simulink model "nms_3Dmodel_inv_wAnkleCPG"  (R2016b)
settings: Solver=ode3  StartTime=0.0  StopTime=tend  FixedStep=ts  RelTol=1e-3  EnableMultiTasking=on
InitFcn:
  | runScripts_inv;
values from neighbouring files (symbols this model uses):
  c = 0.05    [IID_nms_MechInit.m]    (also in nms_MechInit.m)
  c_jointstop = 0.3 / (pi/180)    (= 17.1887338539)    [IID_nms_MechInit.m]    (also in nms_MechInit.m)
  CPG_On = 1    [setCPGPar.m]    (also in setCPGPar_inv.m)
  CtrlPar_FP = [alpha0 alpha_cd alpha_cv]    [setCtrlPar.m]
  CtrlPar_FP_R = [R_hipR0 R_hipR_cd R_hipR_cv]    [setCtrlPar.m]
  CtrlPar_LL = l_clr    [setCtrlPar.m]
  CtrlPar_St = [StPreStim St_M1 St_M2 St_M3 St_M4 St_M5 St_M11]    [setCtrlPar.m]
  CtrlPar_St_R = [R_StPreStim R_St_M1 R_St_M3 R_St_M4]    [setCtrlPar.m]
  CtrlPar_Sw = [SwPreStim SwPhasePari SwPhaseParii SwCtrlPar_H SwCtrlPar_A      SwCtrlPar_Ki SwCtrlPar_Kii SwCtrlPar_Kiii SwCtrlPar_StP]    [setCtrlPar.m]
  CtrlPar_Sw_R = [R_SwPreStim R_Sw_M6]    [setCtrlPar.m]
  CtrlPar_theta0 = parBlCtrl(1)      *1*pi/180    [setCtrlPar.m]
  CtrlPar_Tr = [Tr_St_sup Tr_Sw]    [setCtrlPar.m]
  CtrlPar_Tr_R = [R_Tr_St_sup R_Tr_Sw]    [setCtrlPar.m]
  eref = 0.04    [IID_nms_MechInit.m]    (also in nms_MechInit.m)
  FmaxBFSH = 350    [nms_MechInit.m]
  FmaxGAS = 1500    [IID_nms_MechInit.m]    (also in nms_MechInit.m)
  FmaxGLU = 1500    [IID_nms_MechInit.m]    (also in nms_MechInit.m)
  FmaxHAB = 3000    [nms_MechInit.m]
  FmaxHAD = 4500    [nms_MechInit.m]
  FmaxHAM = 3000    [IID_nms_MechInit.m]    (also in nms_MechInit.m)
  FmaxHFL = 2000    [IID_nms_MechInit.m]    (also in nms_MechInit.m)
  FmaxRF = 1200    [nms_MechInit.m]
  FmaxSOL = 4000    [IID_nms_MechInit.m]    (also in nms_MechInit.m)
  FmaxTA = 800    [IID_nms_MechInit.m]    (also in nms_MechInit.m)
  FmaxVAS = 6000    [IID_nms_MechInit.m]    (also in nms_MechInit.m)
  init_a_tgt = 70*pi/180    (= 1.2217304764)    [setInitPar.m]
  init_a_tgtR = 90*pi/180    (= 1.57079632679)    [setInitPar.m]
  K = 5    [IID_nms_MechInit.m]    (also in nms_MechInit.m)
  leg_l = [D12_T D12_S]    [nms_MechInit.m]
  LongDelay = 0.020    (= 0.02)    [IID_setCtrlPar.m]    (also in nms_MechInit.m = 0.01)
  LongLoopDelay = 0.030    (= 0.03)    [nms_MechInit.m]
  loptBFSH = 0.12    [nms_MechInit.m]
  loptGAS = 0.05    [IID_nms_MechInit.m]    (also in nms_MechInit.m)
  loptGLU = 0.11    [IID_nms_MechInit.m]    (also in nms_MechInit.m)
  loptHAB = 0.09    [nms_MechInit.m]
  loptHAD = 0.10    (= 0.1)    [nms_MechInit.m]
  loptHAM = 0.10    (= 0.1)    [IID_nms_MechInit.m]    (also in nms_MechInit.m)
  loptHFL = 0.11    [IID_nms_MechInit.m]    (also in nms_MechInit.m)
  loptRF = 0.08    [nms_MechInit.m]
  loptSOL = 0.04    [IID_nms_MechInit.m]    (also in nms_MechInit.m)
  loptTA = 0.06    [IID_nms_MechInit.m]    (also in nms_MechInit.m)
  loptVAS = 0.08    [IID_nms_MechInit.m]    (also in nms_MechInit.m)
  lslackBFSH = 0.10    (= 0.1)    [nms_MechInit.m]
  lslackGAS = 0.40    (= 0.4)    [IID_nms_MechInit.m]    (also in nms_MechInit.m)
  lslackGLU = 0.13    [IID_nms_MechInit.m]    (also in nms_MechInit.m)
  lslackHAB = 0.07    [nms_MechInit.m]
  lslackHAD = 0.18    [nms_MechInit.m]
  lslackHAM = 0.31    [IID_nms_MechInit.m]    (also in nms_MechInit.m)
  lslackHFL = 0.10    (= 0.1)    [IID_nms_MechInit.m]    (also in nms_MechInit.m)
  lslackRF = 0.35    [nms_MechInit.m]
  lslackSOL = 0.26    [IID_nms_MechInit.m]    (also in nms_MechInit.m)
  lslackTA = 0.24    [IID_nms_MechInit.m]    (also in nms_MechInit.m)
  lslackVAS = 0.23    [IID_nms_MechInit.m]    (also in nms_MechInit.m)
  massBFSH = 2    [nms_MechInit.m]
  massGAS = 0.45    [IID_nms_MechInit.m]    (also in nms_MechInit.m)
  massGLU = 1.4    [IID_nms_MechInit.m]    (also in nms_MechInit.m)
  massHAB = 1.145    [nms_MechInit.m]
  massHAD = 1.91    [nms_MechInit.m]
  massHAM = 1.82    [IID_nms_MechInit.m]    (also in nms_MechInit.m)
  massHFL = 1.87    [IID_nms_MechInit.m]    (also in nms_MechInit.m)
  massRF = 1    [nms_MechInit.m]
  massSOL = 1.36    [IID_nms_MechInit.m]    (also in nms_MechInit.m)
  massTA = 0.29    [IID_nms_MechInit.m]    (also in nms_MechInit.m)
  massVAS = 2.91    [IID_nms_MechInit.m]    (also in nms_MechInit.m)
  MidDelay = 0.010    (= 0.01)    [IID_setCtrlPar.m]    (also in nms_MechInit.m = 0.005)
  N = 1.5    [IID_nms_MechInit.m]    (also in cmaes_parfor.m = size(x,1); nms_MechInit.m)
  phi12_LowLimit = 70*pi/180    (= 1.2217304764)    [IID_nms_MechInit.m]    (also in nms_MechInit.m)
  phi12_UpLimit = 130*pi/180    (= 2.26892802759)    [IID_nms_MechInit.m]    (also in nms_MechInit.m)
  phi23_UpLimit = 175*pi/180    (= 3.05432619099)    [IID_nms_MechInit.m]    (also in nms_MechInit.m)
  phi34_UpLimit = 230*pi/180    (= 4.01425727959)    [IID_nms_MechInit.m]    (also in nms_MechInit.m)
  phi34R_LowLimit = -15*pi/180    (= -0.261799387799)    [nms_MechInit.m]
  phi34R_UpLimit = 50*pi/180    (= 0.872664625997)    [nms_MechInit.m]
  phimaxGASa = 110*pi/180    (= 1.91986217719)    [IID_nms_MechInit.m]    (also in nms_MechInit.m = 1.74532925199)
  phimaxGASk = 140*pi/180    (= 2.44346095279)    [IID_nms_MechInit.m]    (also in nms_MechInit.m)
  phimaxRFk = 165*pi/180    (= 2.87979326579)    [nms_MechInit.m]
  phimaxSOL = 110*pi/180    (= 1.91986217719)    [IID_nms_MechInit.m]    (also in nms_MechInit.m = 1.74532925199)
  phimaxTA = 80*pi/180    (= 1.3962634016)    [IID_nms_MechInit.m]    (also in nms_MechInit.m)
  phimaxVAS = 165*pi/180    (= 2.87979326579)    [IID_nms_MechInit.m]    (also in nms_MechInit.m)
  phirefBFSH = 160*pi/180    (= 2.79252680319)    [nms_MechInit.m]
  phirefGASa = 80*pi/180    (= 1.3962634016)    [IID_nms_MechInit.m]    (also in nms_MechInit.m)
  phirefGASk = 165*pi/180    (= 2.87979326579)    [IID_nms_MechInit.m]    (also in nms_MechInit.m)
  phirefGLU = 150*pi/180    (= 2.61799387799)    [IID_nms_MechInit.m]    (also in nms_MechInit.m = 2.09439510239)
  phirefHAB = 10*pi/180    (= 0.174532925199)    [nms_MechInit.m]
  phirefHAD = 15*pi/180    (= 0.261799387799)    [nms_MechInit.m]
  phirefHAMh = 155*pi/180    (= 2.70526034059)    [IID_nms_MechInit.m]    (also in nms_MechInit.m = 2.61799387799)
  phirefHAMk = 180*pi/180    (= 3.14159265359)    [IID_nms_MechInit.m]    (also in nms_MechInit.m)
  phirefHFL = 180*pi/180    (= 3.14159265359)    [IID_nms_MechInit.m]    (also in nms_MechInit.m = 2.79252680319)
  phirefRFh = 170*pi/180    (= 2.96705972839)    [nms_MechInit.m]
  phirefRFk = 125*pi/180    (= 2.18166156499)    [nms_MechInit.m]
  phirefSOL = 80*pi/180    (= 1.3962634016)    [IID_nms_MechInit.m]    (also in nms_MechInit.m = 1.57079632679)
  phirefTA = 110*pi/180    (= 1.91986217719)    [IID_nms_MechInit.m]    (also in nms_MechInit.m)
  phirefVAS = 125*pi/180    (= 2.18166156499)    [IID_nms_MechInit.m]    (also in nms_MechInit.m = 2.09439510239)
  phiScaleGASa = acos(rGASamin/rGASamax)/(phiminGASa-phimaxGASa)    [nms_MechInit.m]
  phiScaleGASk = acos(rGASkmin/rGASkmax)/(phiminGASk-phimaxGASk)    [nms_MechInit.m]
  phiScaleRFk = acos(rRFkmin/rRFkmax)/(phiminRFk-phimaxRFk)    [nms_MechInit.m]
  phiScaleSOL = acos(rSOLmin/rSOLmax)/(phiminSOL-phimaxSOL)    [nms_MechInit.m]
  phiScaleTA = acos(rTAmin/rTAmax)/(phiminTA-phimaxTA)    [nms_MechInit.m]
  phiScaleVAS = acos(rVASmin/rVASmax)/(phiminVAS-phimaxVAS)    [nms_MechInit.m]
  rBFSH = 0.04    [nms_MechInit.m]
  rGASamax = 0.06    [nms_MechInit.m]
  rGASkmax = 0.05    [nms_MechInit.m]
  rGLU = 0.10    (= 0.1)    [IID_nms_MechInit.m]    (also in nms_MechInit.m = 0.08)
  rHAB = 0.06    [nms_MechInit.m]
  rHAD = 0.03    [nms_MechInit.m]
  rHAMh = 0.08    [IID_nms_MechInit.m]    (also in nms_MechInit.m)
  rHAMk = 0.05    [IID_nms_MechInit.m]    (also in nms_MechInit.m)
  rHFL = 0.10    (= 0.1)    [IID_nms_MechInit.m]    (also in nms_MechInit.m = 0.08)
  rhoBFSH = 0.7    [nms_MechInit.m]
  rhoGASa = 0.7    [IID_nms_MechInit.m]    (also in nms_MechInit.m)
  rhoGASk = 0.7    [IID_nms_MechInit.m]    (also in nms_MechInit.m)
  rhoGLU = 0.5    [IID_nms_MechInit.m]    (also in nms_MechInit.m)
  rhoHAB = 0.7    [nms_MechInit.m]
  rhoHAD = 1    [nms_MechInit.m]
  rhoHAMh = 0.7    [IID_nms_MechInit.m]    (also in nms_MechInit.m = 0.5)
  rhoHAMk = 0.7    [IID_nms_MechInit.m]    (also in nms_MechInit.m = 0.5)
  rhoHFL = 0.5    [IID_nms_MechInit.m]    (also in nms_MechInit.m)
  rhoRFh = 0.3    [nms_MechInit.m]
  rhoRFk = 0.5    [nms_MechInit.m]
  rhoSOL = 0.5    [IID_nms_MechInit.m]    (also in nms_MechInit.m)
  rhoTA = 0.7    [IID_nms_MechInit.m]    (also in nms_MechInit.m)
  ... (+55 more)
libraries: simulink_extras x30, nmc x30, simulink x22, NMCCPG_Library x13, powerlib_meascontrol x5
(part 6 of 12)

== system nms_3Dmodel_inv_wAnkleCPG/NMC Model/Muscle Actuation Layer/R HFL ==
  note: Excitation Contraction Coupling
  note: HFL Muscle-Tendon Dynamics
  STIM : Inport
  lmtc [m] : Inport  Port=2
  1 : Product  Inputs=**  SaturateOnIntegerOverflow=on  InputSameDT=on  OutDataTypeStr=Inherit: Same as first input
  1/lslack : Gain  Gain=1/lslackHFL  SaturateOnIntegerOverflow=on  OutDataTypeStr=Inherit: Same as input  ParamDataTypeStr=Inherit: Same as input
  2 : Product  Inputs=***  SaturateOnIntegerOverflow=on  InputSameDT=on  OutDataTypeStr=Inherit: Same as first input
  BE force-length relation : Subsystem
  CE force-length relation : Subsystem
  CE inverse force-velocity relation : Subsystem
  Constant : Constant  Value=lslackHFL
  ECC TransferFcn : simulink_extras/Additional Linear/Transfer Fcn (with initial outputs)  N=[1]  D="[tau  1]"  Y0=preA  U0=0
      settings: AttributesFormatString=pre-activation: %<Y0>
  Fmax : Gain  Gain=FmaxHFL  SaturateOnIntegerOverflow=on  OutDataTypeStr=Inherit: Same as input  ParamDataTypeStr=Inherit: Same as input
  Fmax1 : Gain  Gain=FmaxHFL  SaturateOnIntegerOverflow=on  OutDataTypeStr=Inherit: Same as input  ParamDataTypeStr=Inherit: Same as input
  Fv = Fse / (A*Fce) : Product  Inputs=*/  SaturateOnIntegerOverflow=on  InputSameDT=on  OutDataTypeStr=Inherit: Same as first input
  Integrator : Integrator  InitialConditionSource=external  LowerSaturationLimit=0.05  ZeroCross=off
  PE force-length relation : Subsystem
  SE force-length relation : Subsystem
  Sum : Sum  Inputs=|+-  SaturateOnIntegerOverflow=on  InputSameDT=on  OutDataTypeStr=Inherit: Same as first input
  Sum2 : Sum  Inputs=|-+  SaturateOnIntegerOverflow=on  InputSameDT=on  OutDataTypeStr=Inherit: Same as first input
  Sum3 : Sum  SaturateOnIntegerOverflow=on  InputSameDT=on  OutDataTypeStr=Inherit: Same as first input
  Sum4 : Sum  SaturateOnIntegerOverflow=on  InputSameDT=on  OutDataTypeStr=Inherit: Same as first input
  lce/lopt : Gain  Gain=1/loptHFL  SaturateOnIntegerOverflow=on  OutDataTypeStr=Inherit: Same as input  ParamDataTypeStr=Inherit: Same as input
  vmax*lopt : Gain  Gain=vmaxHFL*loptHFL  SaturateOnIntegerOverflow=on  OutDataTypeStr=Inherit: Same as input  ParamDataTypeStr=Inherit: Same as input
  Fmtc : Outport  InitialOutput=0
  Lce : Outport  Port=2  InitialOutput=0
  Vce : Outport  Port=3  InitialOutput=0
  A : Outport  Port=4  InitialOutput=0
  Fac : Outport  Port=5  InitialOutput=0
  wires:
  Fmax1/1 -> Fac/1
  2/1 -> Fmax1/1
  ECC TransferFcn/1 -> 1/2, A/1, 2/2  "A"
  STIM/1 -> ECC TransferFcn/1
  CE inverse force-velocity relation/1(v[vmax]) -> vmax*lopt/1
  Sum3/1 -> Fv = Fse / (A*Fce)/2
  BE force-length relation/1(fbe [Fmax]) -> Sum4/2  "Fbe"
  1/1 -> Sum3/2
  PE force-length relation/1(fpe [Fmax]) -> Sum3/1  "Fpe"
  Sum4/1 -> Fv = Fse / (A*Fce)/1
  CE force-length relation/1(fce [Fmax]) -> 1/1, 2/1  "fl"
  Constant/1 -> Sum2/1
  Sum2/1 -> Integrator/2
  SE force-length relation/1(fse [Fmax]) -> Fmax/1, Sum4/1  "Fse"
  1/lslack/1 -> SE force-length relation/1(lse [lslack])
  Fmax/1 -> Fmtc/1  "Fmtc"
  lmtc [m]/1 -> Sum/1, Sum2/2  "lmtc"
  vmax*lopt/1 -> Vce/1, Integrator/1  "vce"
  Fv = Fse / (A*Fce)/1 -> CE inverse force-velocity relation/1(Fv[Fmax]), 2/3  "fv"
  lce/lopt/1 -> PE force-length relation/1(lce [lopt]), BE force-length relation/1(lce [lopt]), CE force-length relation/1(lce [lopt])
  Sum/1 -> 1/lslack/1  "lse"
  Integrator/1 -> Lce/1, lce/lopt/1, Sum/2  "lce"

== system nms_3Dmodel_inv_wAnkleCPG/NMC Model/Muscle Actuation Layer/R HFL Link ==
  note: HFL Attachment
  phi34 [rad] : Inport
  Constant : Constant  Value=lslackHFL+loptHFL
  Constant1 : Constant  Value=rHFL
  Constant2 : Constant  Value=phirefHFL
  Gain2 : Gain  Gain=rhoHFL
  Product : Product  RndMeth=Zero
  Sum2 : Sum  Inputs=|+-
  Sum5 : Sum  Inputs=|++
  lmtu [m] : Outport
  lever [m] : Outport  Port=2
  wires:
  Gain2/1 -> Sum5/2
  Constant1/1 -> lever [m]/1, Product/2
  Sum2/1 -> Product/1
  Constant2/1 -> Sum2/2
  phi34 [rad]/1 -> Sum2/1
  Product/1 -> Gain2/1
  Sum5/1 -> lmtu [m]/1
  Constant/1 -> Sum5/1

== system nms_3Dmodel_inv_wAnkleCPG/NMC Model/Muscle Actuation Layer/R Hip Roll Joint Limits ==
  note: Ankle Joint Limits
  phi [rad] : Inport
  dphi [rad/s] : Inport  Port=2
  Gain1 : Gain  Gain=c_jointstop
  Gain2 : Gain  Gain=-1
  Gain3 : Gain  Gain=c_jointstop
  Gain4 : Gain  Gain=1/w_max_jointstop
  Limit Ankle Range : simulink/Logic and Bit Operations/Interval Test  IntervalClosedRight=on  uplimit=phi34R_UpLimit + 20*pi/180  IntervalClosedLeft=on  lowlimit=phi34R_LowLimit - 10*pi/180  OutDataTypeStr=boolean
  Logical Operator3 : Logic  Operator=NOT  AllPortsSameDT=off  OutDataTypeStr=boolean
  Mux1 : Mux  Inputs=2
  Mux3 : Mux  Inputs=2
  Overextension Torque : Fcn  Expr="- u(1)  *  (1-u(2)) * (u(2)<1) * (u(1)>0)"
  Overflexion Torque : Fcn  Expr="- u(1)  *  (1-u(2)) * (u(2)<1) * (u(1)<0)"
  Stop Simulation1 : Stop
  Sum : Sum  Inputs=|+-
  Sum1 : Sum  Inputs=|+-
  Sum2 : Sum
  overextension angle : Constant  Value=phi34R_UpLimit
  overflexion angle : Constant  Value=phi34R_LowLimit
  M_stop [Nm] : Outport
  wires:
  Logical Operator3/1 -> Stop Simulation1/1
  Limit Ankle Range/1 -> Logical Operator3/1
  Overextension Torque/1 -> Sum2/1
  Overflexion Torque/1 -> Sum2/2
  Gain2/1 -> Mux3/2
  Sum2/1 -> M_stop [Nm]/1
  Mux1/1 -> Overflexion Torque/1
  overflexion angle/1 -> Sum1/2
  Sum1/1 -> Gain1/1
  Gain1/1 -> Mux1/1
  Gain4/1 -> Mux1/2, Gain2/1
  Sum/1 -> Gain3/1
  phi [rad]/1 -> Limit Ankle Range/1, Sum1/1, Sum/1
  overextension angle/1 -> Sum/2
  dphi [rad/s]/1 -> Gain4/1
  Gain3/1 -> Mux3/1
  Mux3/1 -> Overextension Torque/1

== system nms_3Dmodel_inv_wAnkleCPG/NMC Model/Muscle Actuation Layer/R Knee Joint Limits ==
  note: Ankle Joint Limits
  phi [rad] : Inport
  dphi [rad/s] : Inport  Port=2
  Gain2 : Gain  Gain=-1
  Gain3 : Gain  Gain=c_jointstop
  Gain4 : Gain  Gain=1/w_max_jointstop
  Limit Ankle Range : simulink/Logic and Bit Operations/Interval Test  IntervalClosedRight=on  uplimit=185*pi/180  IntervalClosedLeft=on  lowlimit=40*pi/180  OutDataTypeStr=boolean
  Logical Operator3 : Logic  Operator=NOT  AllPortsSameDT=off  OutDataTypeStr=boolean
  Mux3 : Mux  Inputs=2
  Overextension Torque : Fcn  Expr="- u(1)  *  (1-u(2)) * (u(2)<1) * (u(1)>0)"
  Stop Simulation1 : Stop
  Sum : Sum  Inputs=|+-
  overextension angle : Constant  Value=phi23_UpLimit
  M_stop [Nm] : Outport
  wires:
  Logical Operator3/1 -> Stop Simulation1/1
  Limit Ankle Range/1 -> Logical Operator3/1
  Overextension Torque/1 -> M_stop [Nm]/1
  Gain2/1 -> Mux3/2
  Gain4/1 -> Gain2/1
  Sum/1 -> Gain3/1
  phi [rad]/1 -> Limit Ankle Range/1, Sum/1
  overextension angle/1 -> Sum/2
  dphi [rad/s]/1 -> Gain4/1
  Gain3/1 -> Mux3/1
  Mux3/1 -> Overextension Torque/1

== system nms_3Dmodel_inv_wAnkleCPG/NMC Model/Muscle Actuation Layer/R L Hip Joint Limits ==
  note: Ankle Joint Limits
  phi [rad] : Inport
  dphi [rad/s] : Inport  Port=2
  Gain2 : Gain  Gain=-1
  Gain3 : Gain  Gain=c_jointstop
  Gain4 : Gain  Gain=1/w_max_jointstop
  Limit Ankle Range : simulink/Logic and Bit Operations/Interval Test  IntervalClosedRight=on  uplimit=phi34_UpLimit + 30*pi/180  IntervalClosedLeft=on  lowlimit=10*pi/180  OutDataTypeStr=boolean
  Logical Operator3 : Logic  Operator=NOT  AllPortsSameDT=off  OutDataTypeStr=boolean
  Mux3 : Mux  Inputs=2
  Overextension Torque : Fcn  Expr="- u(1)  *  (1-u(2)) * (u(2)<1) * (u(1)>0)"
  Stop Simulation1 : Stop
  Sum : Sum  Inputs=|+-
  overextension angle : Constant  Value=phi34_UpLimit
  M_stop [Nm] : Outport
  wires:
  Logical Operator3/1 -> Stop Simulation1/1
  Limit Ankle Range/1 -> Logical Operator3/1
  Overextension Torque/1 -> M_stop [Nm]/1
  Gain2/1 -> Mux3/2
  Gain4/1 -> Gain2/1
  Sum/1 -> Gain3/1
  phi [rad]/1 -> Limit Ankle Range/1, Sum/1
  overextension angle/1 -> Sum/2
  dphi [rad/s]/1 -> Gain4/1
  Gain3/1 -> Mux3/1
  Mux3/1 -> Overextension Torque/1

== system nms_3Dmodel_inv_wAnkleCPG/NMC Model/Muscle Actuation Layer/R RF ==
  note: Excitation Contraction Coupling
  note: RF Muscle-Tendon Dynamics
  STIM : Inport
  lmtc [m] : Inport  Port=2
  1 : Product  Inputs=**  SaturateOnIntegerOverflow=on  InputSameDT=on  OutDataTypeStr=Inherit: Same as first input
  1/lslack : Gain  Gain=1/lslackRF  SaturateOnIntegerOverflow=on  OutDataTypeStr=Inherit: Same as input  ParamDataTypeStr=Inherit: Same as input
  2 : Product  Inputs=***  SaturateOnIntegerOverflow=on  InputSameDT=on  OutDataTypeStr=Inherit: Same as first input
  BE force-length relation : Subsystem
  CE force-length relation : Subsystem
  CE inverse force-velocity relation : Subsystem
  Constant : Constant  Value=lslackRF
  ECC TransferFcn : simulink_extras/Additional Linear/Transfer Fcn (with initial outputs)  N=[1]  D="[tau  1]"  Y0=preA  U0=0
      settings: AttributesFormatString=pre-activation: %<Y0>
  Fmax : Gain  Gain=FmaxRF  SaturateOnIntegerOverflow=on  OutDataTypeStr=Inherit: Same as input  ParamDataTypeStr=Inherit: Same as input
  Fmax1 : Gain  Gain=FmaxRF  SaturateOnIntegerOverflow=on  OutDataTypeStr=Inherit: Same as input  ParamDataTypeStr=Inherit: Same as input
  Fv = Fse / (A*Fce) : Product  Inputs=*/  SaturateOnIntegerOverflow=on  InputSameDT=on  OutDataTypeStr=Inherit: Same as first input
  Integrator : Integrator  InitialConditionSource=external  LowerSaturationLimit=0.05  ZeroCross=off
  PE force-length relation : Subsystem
  SE force-length relation : Subsystem
  Sum : Sum  Inputs=|+-  SaturateOnIntegerOverflow=on  InputSameDT=on  OutDataTypeStr=Inherit: Same as first input
  Sum2 : Sum  Inputs=|-+  SaturateOnIntegerOverflow=on  InputSameDT=on  OutDataTypeStr=Inherit: Same as first input
  Sum3 : Sum  SaturateOnIntegerOverflow=on  InputSameDT=on  OutDataTypeStr=Inherit: Same as first input
  Sum4 : Sum  SaturateOnIntegerOverflow=on  InputSameDT=on  OutDataTypeStr=Inherit: Same as first input
  lce/lopt : Gain  Gain=1/loptRF  SaturateOnIntegerOverflow=on  OutDataTypeStr=Inherit: Same as input  ParamDataTypeStr=Inherit: Same as input
  vmax*lopt : Gain  Gain=vmaxRF*loptRF  SaturateOnIntegerOverflow=on  OutDataTypeStr=Inherit: Same as input  ParamDataTypeStr=Inherit: Same as input
  Fmtc : Outport  InitialOutput=0
  Lce : Outport  Port=2  InitialOutput=0
  Vce : Outport  Port=3  InitialOutput=0
  A : Outport  Port=4  InitialOutput=0
  Fac : Outport  Port=5  InitialOutput=0
  wires:
  Fmax1/1 -> Fac/1
  2/1 -> Fmax1/1
  ECC TransferFcn/1 -> A/1, 2/2, 1/2  "fl"
  Fv = Fse / (A*Fce)/1 -> CE inverse force-velocity relation/1(Fv[Fmax]), 2/3  "fv"
  STIM/1 -> ECC TransferFcn/1
  CE inverse force-velocity relation/1(v[vmax]) -> vmax*lopt/1
  Sum3/1 -> Fv = Fse / (A*Fce)/2
  BE force-length relation/1(fbe [Fmax]) -> Sum4/2
  1/1 -> Sum3/2
  PE force-length relation/1(fpe [Fmax]) -> Sum3/1
  Sum4/1 -> Fv = Fse / (A*Fce)/1
  CE force-length relation/1(fce [Fmax]) -> 1/1, 2/1
  Constant/1 -> Sum2/1
  Sum2/1 -> Integrator/2
  SE force-length relation/1(fse [Fmax]) -> Sum4/1, Fmax/1
  1/lslack/1 -> SE force-length relation/1(lse [lslack])
  Fmax/1 -> Fmtc/1  "Fmtc"
  lmtc [m]/1 -> Sum/1, Sum2/2  "lmtc"
  vmax*lopt/1 -> Vce/1, Integrator/1  "vce"
  lce/lopt/1 -> PE force-length relation/1(lce [lopt]), BE force-length relation/1(lce [lopt]), CE force-length relation/1(lce [lopt])
  Sum/1 -> 1/lslack/1  "lse"
  Integrator/1 -> Lce/1, lce/lopt/1, Sum/2  "lce"

== system nms_3Dmodel_inv_wAnkleCPG/NMC Model/Muscle Actuation Layer/R RF Link ==
  note: RF Attachment
  phi34 [rad] : Inport
  phi23 [rad] : Inport  Port=2
  Constant1 : Constant  Value=phimaxRFk
  Constant2 : Constant  Value=phirefRFk
  Constant3 : Constant  Value=rRFh
  Constant4 : Constant  Value=lslackRF+loptRF
  Constant5 : Constant  Value=phirefRFh
  Demux : Demux  Outputs=2
  Gain1 : Gain  Gain=rRFkmax
  Gain2 : Gain  Gain=rhoRFh
  Gain3 : Gain  Gain=phiScaleRFk
  Gain4 : Gain  Gain=rhoRFk/phiScaleRFk
  Gain5 : Gain  Gain=phiScaleRFk
  Mux : Mux  Inputs=2
  Product : Product  RndMeth=Zero
  Sum1 : Sum  Inputs=-+
  Sum2 : Sum  Inputs=|+-
  Sum3 : Sum  Inputs=-+|
  Sum4 : Sum  Inputs=|+-
  Sum5 : Sum  Inputs=++-
  length change term : Trigonometry
  offset correction term : Trigonometry
  variable lever term : Trigonometry  Operator=cos
  lmtu [m] : Outport
  lever34 [m] : Outport  Port=2
  lever23 [m] : Outport  Port=3
  wires:
  Gain5/1 -> offset correction term/1
  Gain3/1 -> length change term/1, variable lever term/1
  Demux/1 -> Gain4/1
  Demux/2 -> lever23 [m]/1
  Gain1/1 -> Demux/1
  Mux/1 -> Gain1/1
  variable lever term/1 -> Mux/2
  Sum1/1 -> Mux/1
  offset correction term/1 -> Sum1/1
  length change term/1 -> Sum1/2
  Constant2/1 -> Sum2/1
  Sum2/1 -> Gain5/1
  Constant1/1 -> Sum2/2, Sum3/1
  Sum3/1 -> Gain3/1
  phi23 [rad]/1 -> Sum3/2
  Product/1 -> Gain2/1
  Constant3/1 -> lever34 [m]/1, Product/2
  Sum4/1 -> Product/1
  Constant5/1 -> Sum4/2
  phi34 [rad]/1 -> Sum4/1
  Gain2/1 -> Sum5/1
  Gain4/1 -> Sum5/3
  Constant4/1 -> Sum5/2
  Sum5/1 -> lmtu [m]/1

== system nms_3Dmodel_inv_wAnkleCPG/NMC Model/Muscle Actuation Layer/R RF1 ==
  note: Excitation Contraction Coupling
  note: RF Muscle-Tendon Dynamics
  STIM : Inport
  lmtc [m] : Inport  Port=2
  1 : Product  Inputs=**  SaturateOnIntegerOverflow=on  InputSameDT=on  OutDataTypeStr=Inherit: Same as first input
  1/lslack : Gain  Gain=1/lslackRF  SaturateOnIntegerOverflow=on  OutDataTypeStr=Inherit: Same as input  ParamDataTypeStr=Inherit: Same as input
  2 : Product  Inputs=***  SaturateOnIntegerOverflow=on  InputSameDT=on  OutDataTypeStr=Inherit: Same as first input
  BE force-length relation : Subsystem
  CE force-length relation : Subsystem
  CE inverse force-velocity relation : Subsystem
  Constant : Constant  Value=lslackRF
  ECC TransferFcn : simulink_extras/Additional Linear/Transfer Fcn (with initial outputs)  N=[1]  D="[tau  1]"  Y0=preA  U0=0
      settings: AttributesFormatString=pre-activation: %<Y0>
  Fmax : Gain  Gain=FmaxRF  SaturateOnIntegerOverflow=on  OutDataTypeStr=Inherit: Same as input  ParamDataTypeStr=Inherit: Same as input
  Fmax1 : Gain  Gain=FmaxRF  SaturateOnIntegerOverflow=on  OutDataTypeStr=Inherit: Same as input  ParamDataTypeStr=Inherit: Same as input
  Fv = Fse / (A*Fce) : Product  Inputs=*/  SaturateOnIntegerOverflow=on  InputSameDT=on  OutDataTypeStr=Inherit: Same as first input
  Integrator : Integrator  InitialConditionSource=external  LowerSaturationLimit=0.05  ZeroCross=off
  PE force-length relation : Subsystem
  SE force-length relation : Subsystem
  Sum : Sum  Inputs=|+-  SaturateOnIntegerOverflow=on  InputSameDT=on  OutDataTypeStr=Inherit: Same as first input
  Sum2 : Sum  Inputs=|-+  SaturateOnIntegerOverflow=on  InputSameDT=on  OutDataTypeStr=Inherit: Same as first input
  Sum3 : Sum  SaturateOnIntegerOverflow=on  InputSameDT=on  OutDataTypeStr=Inherit: Same as first input
  Sum4 : Sum  SaturateOnIntegerOverflow=on  InputSameDT=on  OutDataTypeStr=Inherit: Same as first input
  lce/lopt : Gain  Gain=1/loptRF  SaturateOnIntegerOverflow=on  OutDataTypeStr=Inherit: Same as input  ParamDataTypeStr=Inherit: Same as input
  vmax*lopt : Gain  Gain=vmaxRF*loptRF  SaturateOnIntegerOverflow=on  OutDataTypeStr=Inherit: Same as input  ParamDataTypeStr=Inherit: Same as input
  Fmtc : Outport  InitialOutput=0
  Lce : Outport  Port=2  InitialOutput=0
  Vce : Outport  Port=3  InitialOutput=0
  A : Outport  Port=4  InitialOutput=0
  Fac : Outport  Port=5  InitialOutput=0
  wires:
  Fmax1/1 -> Fac/1
  2/1 -> Fmax1/1
  ECC TransferFcn/1 -> A/1, 2/2, 1/2  "fl"
  Fv = Fse / (A*Fce)/1 -> CE inverse force-velocity relation/1(Fv[Fmax]), 2/3  "fv"
  STIM/1 -> ECC TransferFcn/1
  CE inverse force-velocity relation/1(v[vmax]) -> vmax*lopt/1
  Sum3/1 -> Fv = Fse / (A*Fce)/2
  BE force-length relation/1(fbe [Fmax]) -> Sum4/2
  1/1 -> Sum3/2
  PE force-length relation/1(fpe [Fmax]) -> Sum3/1
  Sum4/1 -> Fv = Fse / (A*Fce)/1
  CE force-length relation/1(fce [Fmax]) -> 1/1, 2/1
  Constant/1 -> Sum2/1
  Sum2/1 -> Integrator/2
  SE force-length relation/1(fse [Fmax]) -> Sum4/1, Fmax/1
  1/lslack/1 -> SE force-length relation/1(lse [lslack])
  Fmax/1 -> Fmtc/1  "Fmtc"
  lmtc [m]/1 -> Sum/1, Sum2/2  "lmtc"
  vmax*lopt/1 -> Vce/1, Integrator/1  "vce"
  lce/lopt/1 -> PE force-length relation/1(lce [lopt]), BE force-length relation/1(lce [lopt]), CE force-length relation/1(lce [lopt])
  Sum/1 -> 1/lslack/1  "lse"
  Integrator/1 -> Lce/1, lce/lopt/1, Sum/2  "lce"

== system nms_3Dmodel_inv_wAnkleCPG/NMC Model/Muscle Actuation Layer/R SOL ==
  note: Excitation Contraction Coupling
  note: SOL Muscle-Tendon Dynamics
  STIM : Inport
  lmtc [m] : Inport  Port=2
  1 : Product  Inputs=**  SaturateOnIntegerOverflow=on  InputSameDT=on  OutDataTypeStr=Inherit: Same as first input
  1/lslack : Gain  Gain=1/lslackSOL  SaturateOnIntegerOverflow=on  OutDataTypeStr=Inherit: Same as input  ParamDataTypeStr=Inherit: Same as input
  2 : Product  Inputs=***  SaturateOnIntegerOverflow=on  InputSameDT=on  OutDataTypeStr=Inherit: Same as first input
  BE force-length relation : Subsystem
  CE force-length relation : Subsystem
  CE inverse force-velocity relation : Subsystem
  Constant : Constant  Value=lslackSOL
  ECC TransferFcn : simulink_extras/Additional Linear/Transfer Fcn (with initial outputs)  N=[1]  D="[tau  1]"  Y0=preA  U0=0
      settings: AttributesFormatString=pre-activation: %<Y0>
  Fmax : Gain  Gain=FmaxSOL  SaturateOnIntegerOverflow=on  OutDataTypeStr=Inherit: Same as input  ParamDataTypeStr=Inherit: Same as input
  Fmax1 : Gain  Gain=FmaxSOL  SaturateOnIntegerOverflow=on  OutDataTypeStr=Inherit: Same as input  ParamDataTypeStr=Inherit: Same as input
  Fv = Fse / (A*Fce) : Product  Inputs=*/  SaturateOnIntegerOverflow=on  InputSameDT=on  OutDataTypeStr=Inherit: Same as first input
  Integrator : Integrator  InitialConditionSource=external  LowerSaturationLimit=0.05  ZeroCross=off
  PE force-length relation : Subsystem
  SE force-length relation : Subsystem
  Sum : Sum  Inputs=|+-  SaturateOnIntegerOverflow=on  InputSameDT=on  OutDataTypeStr=Inherit: Same as first input
  Sum2 : Sum  Inputs=|-+  SaturateOnIntegerOverflow=on  InputSameDT=on  OutDataTypeStr=Inherit: Same as first input
  Sum3 : Sum  SaturateOnIntegerOverflow=on  InputSameDT=on  OutDataTypeStr=Inherit: Same as first input
  Sum4 : Sum  SaturateOnIntegerOverflow=on  InputSameDT=on  OutDataTypeStr=Inherit: Same as first input
  lce/lopt : Gain  Gain=1/loptSOL  SaturateOnIntegerOverflow=on  OutDataTypeStr=Inherit: Same as input  ParamDataTypeStr=Inherit: Same as input
  vmax*lopt : Gain  Gain=vmaxSOL*loptSOL  SaturateOnIntegerOverflow=on  OutDataTypeStr=Inherit: Same as input  ParamDataTypeStr=Inherit: Same as input
  Fmtc : Outport  InitialOutput=0
  Lce : Outport  Port=2  InitialOutput=0
  Vce : Outport  Port=3  InitialOutput=0
  A : Outport  Port=4  InitialOutput=0
  Fac : Outport  Port=5  InitialOutput=0
  wires:
  Fmax1/1 -> Fac/1
  2/1 -> Fmax1/1
  ECC TransferFcn/1 -> 1/2, A/1, 2/2  "A"
  CE force-length relation/1(fce [Fmax]) -> 1/1, 2/1  "fl"
  Fv = Fse / (A*Fce)/1 -> CE inverse force-velocity relation/1(Fv[Fmax]), 2/3  "fv"
  STIM/1 -> ECC TransferFcn/1
  CE inverse force-velocity relation/1(v[vmax]) -> vmax*lopt/1
  Sum3/1 -> Fv = Fse / (A*Fce)/2
  BE force-length relation/1(fbe [Fmax]) -> Sum4/2
  1/1 -> Sum3/2
  PE force-length relation/1(fpe [Fmax]) -> Sum3/1
  Sum4/1 -> Fv = Fse / (A*Fce)/1
  Constant/1 -> Sum2/1
  Sum2/1 -> Integrator/2
  SE force-length relation/1(fse [Fmax]) -> Sum4/1, Fmax/1
  1/lslack/1 -> SE force-length relation/1(lse [lslack])
  Fmax/1 -> Fmtc/1  "Fmtc"
  lmtc [m]/1 -> Sum/1, Sum2/2  "lmtc"
  vmax*lopt/1 -> Vce/1, Integrator/1  "vce"
  lce/lopt/1 -> PE force-length relation/1(lce [lopt]), BE force-length relation/1(lce [lopt]), CE force-length relation/1(lce [lopt])
  Sum/1 -> 1/lslack/1  "lse"
  Integrator/1 -> Lce/1, lce/lopt/1, Sum/2  "lce"

== system nms_3Dmodel_inv_wAnkleCPG/NMC Model/Muscle Actuation Layer/R SOL Link ==
  note: Soleus Attachment
  phi12 [rad] : Inport
  Constant : Constant  Value=lslackSOL+loptSOL
  Constant3 : Constant  Value=phimaxSOL
  Constant5 : Constant  Value=phirefSOL
  Demux1 : Demux  Outputs=2
  Gain2 : Gain  Gain=rSOLmax
  Gain3 : Gain  Gain=phiScaleSOL
  Gain8 : Gain  Gain=phiScaleSOL
  Gain9 : Gain  Gain=rhoSOL/phiScaleSOL
  Mux1 : Mux  Inputs=2
  Sum4 : Sum  Inputs=-+
  Sum5 : Sum  Inputs=|+-
  Sum6 : Sum  Inputs=|+-
  Sum7 : Sum  Inputs=-+|
  length change term1 : Trigonometry
  offset correction term1 : Trigonometry
  variable lever term1 : Trigonometry  Operator=cos
  lmtc [m] : Outport
  lever [m] : Outport  Port=2
  wires:
  Gain8/1 -> offset correction term1/1
  Gain3/1 -> length change term1/1, variable lever term1/1
  Gain2/1 -> Demux1/1
  Mux1/1 -> Gain2/1
  variable lever term1/1 -> Mux1/2
  Sum4/1 -> Mux1/1
  offset correction term1/1 -> Sum4/1
  length change term1/1 -> Sum4/2
  Constant5/1 -> Sum6/1
  Sum6/1 -> Gain8/1
  Constant3/1 -> Sum6/2, Sum7/1
  Sum7/1 -> Gain3/1
  phi12 [rad]/1 -> Sum7/2
  Demux1/2 -> lever [m]/1
  Demux1/1 -> Gain9/1
  Gain9/1 -> Sum5/2
  Sum5/1 -> lmtc [m]/1
  Constant/1 -> Sum5/1

== system nms_3Dmodel_inv_wAnkleCPG/NMC Model/Muscle Actuation Layer/R TA ==
  note: TA Muscle-Tendon Dynamics
  note: Excitation Contraction Coupling
  STIM : Inport
  lmtc [m] : Inport  Port=2
  1 : Product  Inputs=**  SaturateOnIntegerOverflow=on  InputSameDT=on  OutDataTypeStr=Inherit: Same as first input
  1/lslack : Gain  Gain=1/lslackTA  SaturateOnIntegerOverflow=on  OutDataTypeStr=Inherit: Same as input  ParamDataTypeStr=Inherit: Same as input
  2 : Product  Inputs=***  SaturateOnIntegerOverflow=on  InputSameDT=on  OutDataTypeStr=Inherit: Same as first input
  BE force-length relation : Subsystem
  CE force-length relation : Subsystem
  CE inverse force-velocity relation : Subsystem
  Constant : Constant  Value=lslackTA
  ECC TransferFcn : simulink_extras/Additional Linear/Transfer Fcn (with initial outputs)  N=[1]  D="[tau  1]"  Y0=preA  U0=0
      settings: AttributesFormatString=pre-activation: %<Y0>
  Fmax : Gain  Gain=FmaxTA  SaturateOnIntegerOverflow=on  OutDataTypeStr=Inherit: Same as input  ParamDataTypeStr=Inherit: Same as input
  Fmax1 : Gain  Gain=FmaxTA  SaturateOnIntegerOverflow=on  OutDataTypeStr=Inherit: Same as input  ParamDataTypeStr=Inherit: Same as input
  Fv = Fse / (A*Fce) : Product  Inputs=*/  SaturateOnIntegerOverflow=on  InputSameDT=on  OutDataTypeStr=Inherit: Same as first input
  Integrator : Integrator  InitialConditionSource=external  LowerSaturationLimit=0.05  ZeroCross=off
  PE force-length relation : Subsystem
  SE force-length relation : Subsystem
  Sum : Sum  Inputs=|+-  SaturateOnIntegerOverflow=on  InputSameDT=on  OutDataTypeStr=Inherit: Same as first input
  Sum2 : Sum  Inputs=|-+  SaturateOnIntegerOverflow=on  InputSameDT=on  OutDataTypeStr=Inherit: Same as first input
  Sum3 : Sum  SaturateOnIntegerOverflow=on  InputSameDT=on  OutDataTypeStr=Inherit: Same as first input
  Sum4 : Sum  SaturateOnIntegerOverflow=on  InputSameDT=on  OutDataTypeStr=Inherit: Same as first input
  lce/lopt : Gain  Gain=1/loptTA  SaturateOnIntegerOverflow=on  OutDataTypeStr=Inherit: Same as input  ParamDataTypeStr=Inherit: Same as input
  vmax*lopt : Gain  Gain=vmaxTA*loptTA  SaturateOnIntegerOverflow=on  OutDataTypeStr=Inherit: Same as input  ParamDataTypeStr=Inherit: Same as input
  Fmtc : Outport  InitialOutput=0
  Lce : Outport  Port=2  InitialOutput=0
  Vce : Outport  Port=3  InitialOutput=0
  A : Outport  Port=4  InitialOutput=0
  Fac : Outport  Port=5  InitialOutput=0
  wires:
  Fmax1/1 -> Fac/1
  2/1 -> Fmax1/1
  ECC TransferFcn/1 -> A/1, 2/2, 1/2  "A"
  Fv = Fse / (A*Fce)/1 -> CE inverse force-velocity relation/1(Fv[Fmax]), 2/3  "fv"
  STIM/1 -> ECC TransferFcn/1
  Integrator/1 -> Lce/1, Sum/2, lce/lopt/1  "lce"
  Sum/1 -> 1/lslack/1  "lse"
  lce/lopt/1 -> CE force-length relation/1(lce [lopt]), PE force-length relation/1(lce [lopt]), BE force-length relation/1(lce [lopt])
  vmax*lopt/1 -> Vce/1, Integrator/1  "vce"
  lmtc [m]/1 -> Sum2/2, Sum/1  "lmtc"
  Fmax/1 -> Fmtc/1  "Fmtc"
  1/lslack/1 -> SE force-length relation/1(lse [lslack])
  SE force-length relation/1(fse [Fmax]) -> Fmax/1, Sum4/1
  Sum2/1 -> Integrator/2
  Constant/1 -> Sum2/1
  CE force-length relation/1(fce [Fmax]) -> 1/1, 2/1
  Sum4/1 -> Fv = Fse / (A*Fce)/1
  PE force-length relation/1(fpe [Fmax]) -> Sum3/1
  1/1 -> Sum3/2
  BE force-length relation/1(fbe [Fmax]) -> Sum4/2
  Sum3/1 -> Fv = Fse / (A*Fce)/2
  CE inverse force-velocity relation/1(v[vmax]) -> vmax*lopt/1

== system nms_3Dmodel_inv_wAnkleCPG/NMC Model/Muscle Actuation Layer/R TA Link ==
  note: Muscle Length and Moment Arm
  phi12 [rad] : Inport
  Constant : Constant  Value=lslackTA+loptTA
  Constant3 : Constant  Value=phimaxTA
  Constant5 : Constant  Value=phirefTA
  Demux1 : Demux  Outputs=2
  Gain2 : Gain  Gain=rTAmax
  Gain3 : Gain  Gain=phiScaleTA
  Gain8 : Gain  Gain=phiScaleTA
  Gain9 : Gain  Gain=rhoTA/phiScaleTA
  Mux1 : Mux  Inputs=2
  Sum4 : Sum  Inputs=-+
  Sum5 : Sum  Inputs=|++
  Sum6 : Sum  Inputs=|+-
  Sum7 : Sum  Inputs=-+|
  length change term1 : Trigonometry
  offset correction term1 : Trigonometry
  variable lever term1 : Trigonometry  Operator=cos
  lmtc [m] : Outport
  lever [m] : Outport  Port=2
  wires:
  Gain8/1 -> offset correction term1/1
  Gain3/1 -> length change term1/1, variable lever term1/1
  Gain2/1 -> Demux1/1
  Mux1/1 -> Gain2/1
  variable lever term1/1 -> Mux1/2
  Sum4/1 -> Mux1/1
  offset correction term1/1 -> Sum4/1
  length change term1/1 -> Sum4/2
  Constant5/1 -> Sum6/1
  Sum6/1 -> Gain8/1
  Constant3/1 -> Sum6/2, Sum7/1
  Sum7/1 -> Gain3/1
  phi12 [rad]/1 -> Sum7/2
  Demux1/2 -> lever [m]/1
  Demux1/1 -> Gain9/1
  Gain9/1 -> Sum5/2
  Sum5/1 -> lmtc [m]/1
  Constant/1 -> Sum5/1

== system nms_3Dmodel_inv_wAnkleCPG/NMC Model/Muscle Actuation Layer/R VAS ==
  note: Excitation Contraction Coupling
  note: VAS Muscle-Tendon Dynamics
  STIM : Inport
  lmtc [m] : Inport  Port=2
  1 : Product  Inputs=**  SaturateOnIntegerOverflow=on  InputSameDT=on  OutDataTypeStr=Inherit: Same as first input
  1/lslack : Gain  Gain=1/lslackVAS  SaturateOnIntegerOverflow=on  OutDataTypeStr=Inherit: Same as input  ParamDataTypeStr=Inherit: Same as input
  2 : Product  Inputs=***  SaturateOnIntegerOverflow=on  InputSameDT=on  OutDataTypeStr=Inherit: Same as first input
  BE force-length relation : Subsystem
  CE force-length relation : Subsystem
  CE inverse force-velocity relation : Subsystem
  Constant : Constant  Value=lslackVAS
  ECC TransferFcn : simulink_extras/Additional Linear/Transfer Fcn (with initial outputs)  N=[1]  D="[tau  1]"  Y0=preA  U0=0
      settings: AttributesFormatString=pre-activation: %<Y0>
  Fmax : Gain  Gain=FmaxVAS  SaturateOnIntegerOverflow=on  OutDataTypeStr=Inherit: Same as input  ParamDataTypeStr=Inherit: Same as input
  Fmax1 : Gain  Gain=FmaxVAS  SaturateOnIntegerOverflow=on  OutDataTypeStr=Inherit: Same as input  ParamDataTypeStr=Inherit: Same as input
  Fv = Fse / (A*Fce) : Product  Inputs=*/  SaturateOnIntegerOverflow=on  InputSameDT=on  OutDataTypeStr=Inherit: Same as first input
  Integrator : Integrator  InitialConditionSource=external  LowerSaturationLimit=0.05  ZeroCross=off
  PE force-length relation : Subsystem
  SE force-length relation : Subsystem
  Sum : Sum  Inputs=|+-  SaturateOnIntegerOverflow=on  InputSameDT=on  OutDataTypeStr=Inherit: Same as first input
  Sum2 : Sum  Inputs=|-+  SaturateOnIntegerOverflow=on  InputSameDT=on  OutDataTypeStr=Inherit: Same as first input
  Sum3 : Sum  SaturateOnIntegerOverflow=on  InputSameDT=on  OutDataTypeStr=Inherit: Same as first input
  Sum4 : Sum  SaturateOnIntegerOverflow=on  InputSameDT=on  OutDataTypeStr=Inherit: Same as first input
  lce/lopt : Gain  Gain=1/loptVAS  SaturateOnIntegerOverflow=on  OutDataTypeStr=Inherit: Same as input  ParamDataTypeStr=Inherit: Same as input
  vmax*lopt : Gain  Gain=vmaxVAS*loptVAS  SaturateOnIntegerOverflow=on  OutDataTypeStr=Inherit: Same as input  ParamDataTypeStr=Inherit: Same as input
  Fmtc : Outport  InitialOutput=0
  Lce : Outport  Port=2  InitialOutput=0
  Vce : Outport  Port=3  InitialOutput=0
  A : Outport  Port=4  InitialOutput=0
  Fac : Outport  Port=5  InitialOutput=0
  wires:
  Fmax1/1 -> Fac/1
  2/1 -> Fmax1/1
  ECC TransferFcn/1 -> A/1, 2/2, 1/2  "fl"
  Fv = Fse / (A*Fce)/1 -> CE inverse force-velocity relation/1(Fv[Fmax]), 2/3  "fv"
  STIM/1 -> ECC TransferFcn/1
  CE inverse force-velocity relation/1(v[vmax]) -> vmax*lopt/1
  Sum3/1 -> Fv = Fse / (A*Fce)/2
  BE force-length relation/1(fbe [Fmax]) -> Sum4/2
  1/1 -> Sum3/2
  PE force-length relation/1(fpe [Fmax]) -> Sum3/1
  Sum4/1 -> Fv = Fse / (A*Fce)/1
  CE force-length relation/1(fce [Fmax]) -> 1/1, 2/1
  Constant/1 -> Sum2/1
  Sum2/1 -> Integrator/2
  SE force-length relation/1(fse [Fmax]) -> Sum4/1, Fmax/1
  1/lslack/1 -> SE force-length relation/1(lse [lslack])
  Fmax/1 -> Fmtc/1  "Fmtc"
  lmtc [m]/1 -> Sum/1, Sum2/2  "lmtc"
  vmax*lopt/1 -> Vce/1, Integrator/1  "vce"
  lce/lopt/1 -> PE force-length relation/1(lce [lopt]), BE force-length relation/1(lce [lopt]), CE force-length relation/1(lce [lopt])
  Sum/1 -> 1/lslack/1  "lse"
  Integrator/1 -> Lce/1, lce/lopt/1, Sum/2  "lce"

== system nms_3Dmodel_inv_wAnkleCPG/NMC Model/Muscle Actuation Layer/R VAS Link ==
  note: Muscle Length and Moment Arm
  phi23 [rad] : Inport
  Constant : Constant  Value=lslackVAS+loptVAS
  Constant1 : Constant  Value=phimaxVAS
  Constant2 : Constant  Value=phirefVAS
  Demux : Demux  Outputs=2
  Gain1 : Gain  Gain=rVASmax
  Gain3 : Gain  Gain=phiScaleVAS
  Gain4 : Gain  Gain=rhoVAS/phiScaleVAS
  Gain5 : Gain  Gain=phiScaleVAS
  Mux : Mux  Inputs=2
  Sum1 : Sum  Inputs=-+
  Sum2 : Sum  Inputs=|+-
  Sum3 : Sum  Inputs=-+|
  Sum5 : Sum  Inputs=|+-
  length change term : Trigonometry
  offset correction term : Trigonometry
  variable lever term : Trigonometry  Operator=cos
  lmtu [m] : Outport
  lever [m] : Outport  Port=2
  wires:
  Gain4/1 -> Sum5/2
  Gain5/1 -> offset correction term/1
  Gain3/1 -> length change term/1, variable lever term/1
  Demux/1 -> Gain4/1
  Demux/2 -> lever [m]/1
  Gain1/1 -> Demux/1
  Mux/1 -> Gain1/1
  variable lever term/1 -> Mux/2
  Sum1/1 -> Mux/1
  offset correction term/1 -> Sum1/1
  length change term/1 -> Sum1/2
  Constant2/1 -> Sum2/1
  Sum2/1 -> Gain5/1
  Constant1/1 -> Sum2/2, Sum3/1
  Sum3/1 -> Gain3/1
  phi23 [rad]/1 -> Sum3/2
  Sum5/1 -> lmtu [m]/1
  Constant/1 -> Sum5/1

== system nms_3Dmodel_inv_wAnkleCPG/NMC Model/Neural Control Layer (Spinal Cord Control)/L Stance Phase (coronal) ==
  note: M4: compensate swing leg
  note: M3: balance trunk
  note: Left Stance Phase Control
  CtrlPar : Inport
  theta_tgt [rad] : Inport  Port=2
  theta dtheta [rad rad/s] : Inport  Port=3
  CSwingStim : Inport  Port=4
  FmHAB : Inport  Port=5
  Enable : EnablePort  StatesWhenEnabling=reset  ZeroCross=off
  Demux1 : Demux  Outputs=2
  Demux2 : Demux
  Demux7 : Demux  Outputs=2
  Demux8 : Demux  Outputs=2
  Divide{1,4,6..7,9,14..15} (7 alike) : Product
  Gain2 : Gain  Gain=-1
  Gain3 : Gain  Gain=-1
  Mux1 : Mux  Inputs=2
  Mux2 : Mux  Inputs=2
  R_parSt_M1 : Selector  InputPortWidth=R_St_i  IndexOptions=Index vector (dialog)  Indices=R_parSt_M1_i  OutputSizes=1
  R_parSt_M3 : Selector  InputPortWidth=R_St_i  IndexOptions=Index vector (dialog)  Indices=R_parSt_M3_i  OutputSizes=1
  R_parSt_M4 : Selector  InputPortWidth=R_St_i  IndexOptions=Index vector (dialog)  Indices=R_parSt_M4_i  OutputSizes=1
  R_parSt_PreS : Selector  InputPortWidth=R_St_i  IndexOptions=Index vector (dialog)  Indices=R_parSt_PreS_i  OutputSizes=1
  Sum4 : Sum  Inputs=-+|  SaturateOnIntegerOverflow=on  InputSameDT=on  OutDataTypeStr=Inherit: Same as first input
  Sum5 : Sum  Inputs=|++  SaturateOnIntegerOverflow=on  InputSameDT=on  OutDataTypeStr=Inherit: Same as first input
  Sum6 : Sum  Inputs=|++  SaturateOnIntegerOverflow=on  InputSameDT=on  OutDataTypeStr=Inherit: Same as first input
  positive half1 : Saturate  UpperLimit=inf  LowerLimit=0  ZeroCross=off
  positive half2 : Saturate  UpperLimit=inf  LowerLimit=0  ZeroCross=off
  S_0_St : Outport  OutputWhenDisabled=reset  InitialOutput=0
  S_M1 [HAB] : Outport  Port=2  OutputWhenDisabled=reset  InitialOutput=0
  S_M3 [HAB HAD] : Outport  Port=3  OutputWhenDisabled=reset  InitialOutput=0
  S_M4 [HAB HAD] : Outport  Port=4  OutputWhenDisabled=reset  InitialOutput=0
  wires:
  FmHAB/1 -> Divide7/2
  Divide7/1 -> S_M1 [HAB]/1  "HAB"
  R_parSt_M1/1 -> Divide7/1  "FGain_HAB"
  positive half2/1 -> Mux1/2
  positive half1/1 -> Mux1/1
  Divide1/1 -> Mux2/2  "HAD"
  Demux1/2 -> Divide1/1  "SGainCHAD_HAD"
  Divide9/1 -> Mux2/1  "HAB"
  Demux1/1 -> Divide9/1  "SGainCHAB_HAB"
  R_parSt_M4/1 -> Demux1/1
  Demux8/2 -> Divide1/2  "Stim_CHAD"
  Demux8/1 -> Divide9/2  "Stim_CHAB"
  Mux2/1 -> S_M4 [HAB HAD]/1
  CSwingStim/1 -> Demux8/1
  R_parSt_M3/1 -> Demux2/1
  CtrlPar/1 -> R_parSt_M1/1, R_parSt_M3/1, R_parSt_M4/1, R_parSt_PreS/1
  R_parSt_PreS/1 -> S_0_St/1
  Mux1/1 -> S_M3 [HAB HAD]/1
  Sum6/1 -> positive half2/1  "HAD"
  Sum5/1 -> positive half1/1  "HAB"
  Divide15/1 -> Sum6/2
  Divide14/1 -> Sum6/1
  Divide6/1 -> Sum5/2
  Divide4/1 -> Sum5/1
  Gain3/1 -> Divide6/1
  Gain2/1 -> Divide4/1
  Demux2/4 -> Divide15/2  "GainDTh_HAD"
  Demux2/3 -> Divide14/2  "GainTh_HAD"
  Demux2/2 -> Divide6/2  "GainDTh_HAB"
  Demux2/1 -> Divide4/2  "GainTh_HAB"
  Sum4/1 -> Divide14/1, Gain2/1
  theta_tgt [rad]/1 -> Sum4/1
  Demux7/2 -> Divide15/1, Gain3/1  "dtheta"
  Demux7/1 -> Sum4/2  "theta"
  theta dtheta [rad rad/s]/1 -> Demux7/1

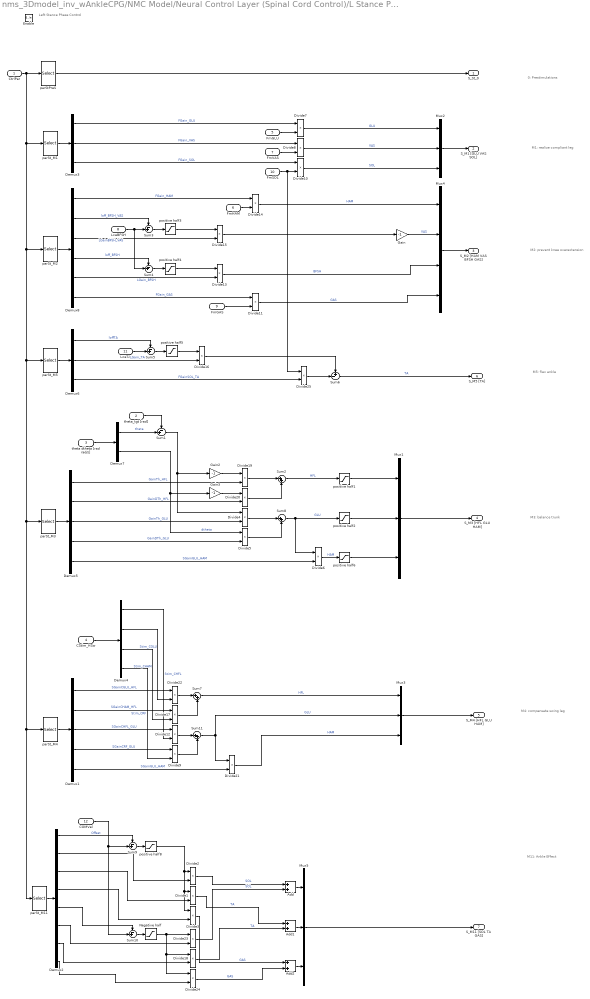
== system nms_3Dmodel_inv_wAnkleCPG/NMC Model/Neural Control Layer (Spinal Cord Control)/L Stance Phase (sagittal) ==
  note: M11: Ankle Effect
  note: M4: compensate swing leg
  note: M3: balance trunk
  note: M5: flex ankle
  note: M2: prevent knee overextension
  note: M1: realize compliant leg
  note: 0: Prestimulations
  note: Left Stance Phase Control
  CtrlPar : Inport
  theta_tgt [rad] : Inport  Port=2
  theta dtheta [rad rad/s] : Inport  Port=3
  CStim_HSw : Inport  Port=4
  FmGLU : Inport  Port=5
  FmHAM : Inport  Port=6
  FmVAS : Inport  Port=7
  LceBFSH : Inport  Port=8
  FmGAS : Inport  Port=9
  FmSOL : Inport  Port=10
  LceTA : Inport  Port=11
  COMVel : Inport  Port=12
  Enable : EnablePort  StatesWhenEnabling=reset  ZeroCross=off
  Add : Sum
  Add1 : Sum
  Add2 : Sum
  Demux1 : Demux  Outputs=5
  Demux2 : Demux  Outputs=8
  Demux3 : Demux  Outputs=3
  Demux4 : Demux
  Demux5 : Demux  Outputs=5
  Demux6 : Demux  Outputs=3
  Demux7 : Demux  Outputs=2
  Demux8 : Demux  Outputs=6
  Divide{1..25} (25 alike) : Product
  Gain : Gain  Gain=-1
  Gain2 : Gain  Gain=-1
  Gain3 : Gain  Gain=-1
  Mux{1..3,5} (4 alike) : Mux  Inputs=3
  Mux4 : Mux
  Negative half : Saturate  UpperLimit=0  LowerLimit=-inf  ZeroCross=off
  Sum{1,3..5,9..10} (6 alike) : Sum  Inputs=-+|  SaturateOnIntegerOverflow=on  InputSameDT=on  OutDataTypeStr=Inherit: Same as first input
  Sum{2,7..8,11} (4 alike) : Sum  Inputs=|++  SaturateOnIntegerOverflow=on  InputSameDT=on  OutDataTypeStr=Inherit: Same as first input
  Sum6 : Sum  Inputs=+-|  SaturateOnIntegerOverflow=on  InputSameDT=on  OutDataTypeStr=Inherit: Same as first input
  parStPreS : Selector  InputPortWidth=St_i  IndexOptions=Index vector (dialog)  Indices=parSt_PreS_i  OutputSizes=1
  parSt_M1 : Selector  InputPortWidth=St_i  IndexOptions=Index vector (dialog)  Indices=parSt_M1_i  OutputSizes=1
  parSt_M11 : Selector  InputPortWidth=St_i  IndexOptions=Index vector (dialog)  Indices=parSt_M11_i  OutputSizes=1
  parSt_M2 : Selector  InputPortWidth=St_i  IndexOptions=Index vector (dialog)  Indices=parSt_M2_i  OutputSizes=1
  parSt_M3 : Selector  InputPortWidth=St_i  IndexOptions=Index vector (dialog)  Indices=parSt_M3_i  OutputSizes=1
  parSt_M4 : Selector  InputPortWidth=St_i  IndexOptions=Index vector (dialog)  Indices=parSt_M4_i  OutputSizes=1
  parSt_M5 : Selector  InputPortWidth=St_i  IndexOptions=Index vector (dialog)  Indices=parSt_M5_i  OutputSizes=1
  positive half{1..6,8} (7 alike) : Saturate  UpperLimit=inf  LowerLimit=0  ZeroCross=off
  S_St_0 : Outport  OutputWhenDisabled=reset  InitialOutput=0
  S_M1 [GLU VAS SOL] : Outport  Port=2  OutputWhenDisabled=reset  InitialOutput=0
  S_M2 [HAM VAS BFSH GAS] : Outport  Port=3  OutputWhenDisabled=reset  InitialOutput=0
  S_M3 [HFL GLU HAM] : Outport  Port=4  OutputWhenDisabled=reset  InitialOutput=0
  S_M4 [HFL GLU HAM] : Outport  Port=5  OutputWhenDisabled=reset  InitialOutput=0
  S_M5 [TA] : Outport  Port=6  OutputWhenDisabled=reset  InitialOutput=0
  S_M11 [SOL TA GAS] : Outport  Port=7  OutputWhenDisabled=reset  InitialOutput=0
  wires:
  Demux2/1 -> Sum9/1  "Offset"
  positive half8/1 -> Divide2/1, Divide1/1, Divide3/1
  Negative half/1 -> Divide24/1, Divide18/1, Divide23/1
  Sum10/1 -> Negative half/1
  Demux2/2 -> Divide2/2
  Mux5/1 -> S_M11 [SOL TA GAS]/1
  Divide3/1 -> Add2/1  "GAS"
  Divide1/1 -> Add1/1  "TA"
  Divide2/1 -> Add/1  "SOL"
  Sum9/1 -> positive half8/1
  COMVel/1 -> Sum10/2, Sum9/2
  parSt_M11/1 -> Demux2/1
  Divide9/1 -> Sum11/2
  Sum11/1 -> Divide21/1, Mux3/2  "GLU"
  Divide12/1 -> Sum11/1
  Divide17/1 -> Sum7/2
  Sum7/1 -> Mux3/1  "HFL"
  Divide22/1 -> Sum7/1
  Demux1/4 -> Divide9/1  "SGainCRF_GLU"
  Demux1/2 -> Divide17/1  "SGainCHAM_HFL"
  Demux4/4 -> Divide9/2  "Stim_CRF"
  Demux4/3 -> Divide17/2  "Stim_CHAM"
  Divide21/1 -> Mux3/3  "HAM"
  Demux1/5 -> Divide21/2  "SGainGLU_HAM"
  Mux3/1 -> S_M4 [HFL GLU HAM]/1
  Demux4/2 -> Divide22/2  "Stim_CGLU"
  Demux4/1 -> Divide12/2  "Stim_CHFL"
  CStim_HSw/1 -> Demux4/1
  Demux1/3 -> Divide12/1  "SGainCHFL_GLU"
  Demux1/1 -> Divide22/1  "SGainCGLU_HFL"
  parSt_M4/1 -> Demux1/1
  positive half6/1 -> Mux1/3
  positive half2/1 -> Mux1/2
  positive half1/1 -> Mux1/1
  theta_tgt [rad]/1 -> Sum1/1
  Divide6/1 -> positive half6/1  "HAM"
  Demux5/5 -> Divide6/2  "SGainGLU_HAM"
  Mux1/1 -> S_M3 [HFL GLU HAM]/1
  Sum8/1 -> positive half2/1, Divide6/1  "GLU"
  Sum2/1 -> positive half1/1  "HFL"
  Divide5/1 -> Sum8/2
  Divide4/1 -> Sum8/1
  Divide20/1 -> Sum2/2
  Divide19/1 -> Sum2/1
  Gain3/1 -> Divide20/1
  Gain2/1 -> Divide19/1
  Sum1/1 -> Divide4/1, Gain2/1
  Demux7/2 -> Divide5/1, Gain3/1  "dtheta"
  Demux7/1 -> Sum1/2  "theta"
  theta dtheta [rad rad/s]/1 -> Demux7/1
  Demux5/4 -> Divide5/2  "GainDTh_GLU"
  Demux5/3 -> Divide4/2  "GainTh_GLU"
  Demux5/2 -> Divide20/2  "GainDTh_HFL"
  Demux5/1 -> Divide19/2  "GainTh_HFL"
  parSt_M3/1 -> Demux5/1
  Mux4/1 -> S_M2 [HAM VAS BFSH GAS]/1
  LceTA/1 -> Sum5/2
  Sum6/1 -> S_M5 [TA]/1  "TA"
  Demux6/3 -> Divide25/2  "FGainSOL_TA"
  Demux6/2 -> Divide16/2  "LGain_TA"
  Demux6/1 -> Sum5/1  "loffTA"
  parSt_M5/1 -> Demux6/1
  Divide25/1 -> Sum6/2
  Divide16/1 -> Sum6/1
  positive half5/1 -> Divide16/1
  Sum5/1 -> positive half5/1
  FmGAS/1 -> Divide11/2
  LceBFSH/1 -> Sum4/2, Sum3/2
  FmHAM/1 -> Divide14/2
  Demux8/4 -> Sum4/1  "loff_BFSH"
  positive half4/1 -> Divide13/1
  Sum4/1 -> positive half4/1
  Gain/1 -> Mux4/2  "VAS"
  Divide14/1 -> Mux4/1  "HAM"
  Demux8/1 -> Divide14/1  "FGain_HAM"
  Divide11/1 -> Mux4/4  "GAS"
  Divide13/1 -> Mux4/3  "BFSH"
  Divide15/1 -> Gain/1
  Demux8/2 -> Sum3/1  "loff_BFSH_VAS"
  positive half3/1 -> Divide15/1
  Demux8/6 -> Divide11/1  "FGain_GAS"
  Demux8/5 -> Divide13/2  "LGain_BFSH"
  Demux8/3 -> Divide15/2  "LGainBFSH_VAS"
  Sum3/1 -> positive half3/1
  parSt_M2/1 -> Demux8/1
  FmSOL/1 -> Divide25/1, Divide10/2
  FmVAS/1 -> Divide8/2
  FmGLU/1 -> Divide7/2
  Mux2/1 -> S_M1 [GLU VAS SOL]/1
  Divide7/1 -> Mux2/1  "GLU"
  Demux3/1 -> Divide7/1  "FGain_GLU"
  Divide8/1 -> Mux2/2  "VAS"
  Divide10/1 -> Mux2/3  "SOL"
  Demux3/3 -> Divide10/1  "FGain_SOL"
  Demux3/2 -> Divide8/1  "FGain_VAS"
  parSt_M1/1 -> Demux3/1
  parStPreS/1 -> S_St_0/1
  CtrlPar/1 -> parSt_M4/1, parSt_M11/1, parSt_M3/1, parSt_M5/1, parSt_M2/1, parSt_M1/1, parStPreS/1
  Demux2/3 -> Divide1/2
  Demux2/4 -> Divide3/2
  Demux2/5 -> Sum10/1
  Divide24/1 -> Add2/2  "GAS"
  Divide18/1 -> Add1/2  "TA"
  Divide23/1 -> Add/2  "SOL"
  Demux2/6 -> Divide23/2
  Demux2/7 -> Divide18/2
  Demux2/8 -> Divide24/2
  Add/1 -> Mux5/1
  Add1/1 -> Mux5/2
  Add2/1 -> Mux5/3
